simulink model "tyre"  (R2022b)
settings: Solver=ode4  StartTime=0.0  StopTime=simin.Time.data(end)  FixedStep=0.001  RelTol=1e-3
model workspace (MAT data in the model file):
  Fz_stat_FL = Simulink.Parameter
  Fz_stat_FL.Value = 3921.3656
  Fz_stat_FL.DataType = 'double'
  Fz_stat_FL.DocUnits = 'N'
  Fz_stat_FL.Complexity = 'real'
  Fz_stat_FL.Dimensions = [1 1]
  Fz_stat_FR = Simulink.Parameter
  Fz_stat_FR.Value = 3921.3656
  Fz_stat_FR.DataType = 'double'
  Fz_stat_FR.DocUnits = 'N'
  Fz_stat_FR.Complexity = 'real'
  Fz_stat_FR.Dimensions = [1 1]
  Fz_stat_RL = Simulink.Parameter
  Fz_stat_RL.Value = 3922.1269
  Fz_stat_RL.DataType = 'double'
  Fz_stat_RL.DocUnits = 'N'
  Fz_stat_RL.Complexity = 'real'
  Fz_stat_RL.Dimensions = [1 1]
  Fz_stat_RR = Simulink.Parameter
  Fz_stat_RR.Value = 3922.1267
  Fz_stat_RR.DataType = 'double'
  Fz_stat_RR.DocUnits = 'N'
  Fz_stat_RR.Complexity = 'real'
  Fz_stat_RR.Dimensions = [1 1]
  cog_height = Simulink.Parameter
  cog_height.Value = 0.604
  cog_height.DataType = 'double'
  cog_height.DocUnits = 'm'
  cog_height.Complexity = 'real'
  cog_height.Dimensions = [1 1]
  g = Simulink.Parameter
  g.Value = 9.806
  g.DataType = 'double'
  g.DocUnits = 'm/s^2'
  g.Complexity = 'real'
  g.Dimensions = [1 1]
  lF = Simulink.Parameter
  lF.Value = 1.466
  lF.DataType = 'double'
  lF.DocUnits = 'm'
  lF.Complexity = 'real'
  lF.Dimensions = [1 1]
  lR = Simulink.Parameter
  lR.Value = 1.509
  lR.DataType = 'double'
  lR.DocUnits = 'm'
  lR.Complexity = 'real'
  lR.Dimensions = [1 1]
  pitchAngle = Simulink.Parameter
  pitchAngle.Value = [0.00443372596055 0.00472012698538 0.00500652801021 0.00529292903504 0.00557933005986 0.00586573108469 0.00615213210952 0.00643853313435 0.00672493415917 0.007011335184 0.00729773620883 0.00758413723366 ... (200 elements, 1x200)]
  pitchAngle.DataType = 'double'
  pitchAngle.DocUnits = 'rad'
  pitchAngle.Complexity = 'real'
  pitchAngle.Dimensions = [1 200]
  pitchStiffness = Simulink.Parameter
  pitchStiffness.Value = [286621.759635 286644.842257 286407.773968 286374.136656 286600.567598 286901.705993 287109.32323 287190.659823 287245.018359 287344.728913 287488.533524 287631.863692 ... (200 elements, 1x200)]
  pitchStiffness.DataType = 'double'
  pitchStiffness.DocUnits = 'N*m*s/rad'
  pitchStiffness.Complexity = 'real'
  pitchStiffness.Dimensions = [1 200]
  pitch_inertia = Simulink.Parameter
  pitch_inertia.Value = 2180.5
  pitch_inertia.DataType = 'double'
  pitch_inertia.DocUnits = 'kg * m^2'
  pitch_inertia.Complexity = 'real'
  pitch_inertia.Dimensions = [1 1]
  pitching_coefficient = Simulink.Parameter
  pitching_coefficient.Value = -0.002
  pitching_coefficient.DataType = 'double'
  pitching_coefficient.DocUnits = '1'
  pitching_coefficient.Complexity = 'real'
  pitching_coefficient.Dimensions = [1 1]
  rdyn = Simulink.Parameter
  rdyn.Value = 0.309
  rdyn.DataType = 'double'
  rdyn.DocUnits = 'm'
  rdyn.Complexity = 'real'
  rdyn.Dimensions = [1 1]
  reference_area = Simulink.Parameter
  reference_area.Value = 2.4
  reference_area.DataType = 'double'
  reference_area.DocUnits = 'm^2'
  reference_area.Complexity = 'real'
  reference_area.Dimensions = [1 1]
  rho = Simulink.Parameter
  rho.Value = 1.2
  rho.DataType = 'double'
  rho.DocUnits = 'kg / m^3'
  rho.Complexity = 'real'
  rho.Dimensions = [1 1]
  rollStiffness_F = Simulink.Parameter
  rollStiffness_F.Value = -66168.4036
  rollStiffness_F.DataType = 'double'
  rollStiffness_F.DocUnits = 'N*m/rad'
  rollStiffness_F.Complexity = 'real'
  rollStiffness_F.Dimensions = [1 1]
  rollStiffness_R = Simulink.Parameter
  rollStiffness_R.Value = -79058.3706
  rollStiffness_R.DataType = 'double'
  rollStiffness_R.DocUnits = 'N*m/rad'
  rollStiffness_R.Complexity = 'real'
  rollStiffness_R.Dimensions = [1 1]
  sprung_mass = Simulink.Parameter
  sprung_mass.Value = 1373.3
  sprung_mass.DataType = 'double'
  sprung_mass.DocUnits = 'kg'
  sprung_mass.Complexity = 'real'
  sprung_mass.Dimensions = [1 1]
  tire = Simulink.Parameter
  tire.Value.MDI_Header.FILE_VERSION = 2
  tire.Value.Model.USE_MODE = 14
  tire.Value.Dim.UNLOADED_RADIUS = 0.3185
  tire.Value.Dim.WIDTH = 0.205
  tire.Value.Dim.RIM_RADIUS = 0.1905
  tire.Value.Dim.RIM_WIDTH = 0.1524
  tire.Value.Dim.ASPECT_RATIO = 0.6
  tire.Value.Vertical.VERTICAL_STIFFNESS = 236700
  tire.Value.Vertical.VERTICAL_DAMPING = 50
  tire.Value.Vertical.BREFF = 5
  tire.Value.Vertical.DREFF = 0.3
  tire.Value.Vertical.FREFF = 0.1
  tire.Value.Vertical.FNOMIN = 6500
  tire.Value.Range.KPUMIN = -0.3
  tire.Value.Range.KPUMAX = 0.3
  tire.Value.Range.ALPMIN = -0.1745
  tire.Value.Range.ALPMAX = 0.1745
  tire.Value.Range.CAMMIN = -0.1047
  tire.Value.Range.CAMMAX = 0.1047
  tire.Value.Range.FZMIN = 400
  tire.Value.Range.FZMAX = 8500
  tire.Value.Scale.LFZO = 1
  tire.Value.Scale.LCX = 1
  tire.Value.Scale.LMUX = 1
  tire.Value.Scale.LEX = 1
  tire.Value.Scale.LKX = 1
  tire.Value.Scale.LHX = 1
  tire.Value.Scale.LVX = 1
  tire.Value.Scale.LGAX = 1
  tire.Value.Scale.LCY = 1
  tire.Value.Scale.LMUY = 1
  tire.Value.Scale.LEY = 1
  tire.Value.Scale.LKY = 1
  tire.Value.Scale.LHY = 1
  tire.Value.Scale.LVY = 1
  tire.Value.Scale.LGAY = 1
  tire.Value.Scale.LTR = 1
  tire.Value.Scale.LRES = 1
  tire.Value.Scale.LGAZ = 1
  tire.Value.Scale.LXAL = 1
  tire.Value.Scale.LYKA = 1
  tire.Value.Scale.LVYKA = 1
  tire.Value.Scale.LS = 1
  tire.Value.Scale.LSGKP = 1
  tire.Value.Scale.LSGAL = 1
  tire.Value.Scale.LGYR = 1
  tire.Value.Scale.LMX = 1
  tire.Value.Scale.LVMX = 1
  tire.Value.Scale.LMY = 1
  tire.Value.Long.PCX1 = 1.6055
  tire.Value.Long.PDX1 = 1.1703
  tire.Value.Long.PDX2 = -0.081328
  tire.Value.Long.PDX3 = 0
  tire.Value.Long.PEX1 = 0.53409
  tire.Value.Long.PEX2 = -0.019956
  tire.Value.Long.PEX3 = 0.18089
  tire.Value.Long.PEX4 = 2.9951e-07
  tire.Value.Long.PKX1 = 36.411
  tire.Value.Long.PKX2 = 0.12615
  tire.Value.Long.PKX3 = 0.51289
  tire.Value.Long.PHX1 = 0
  tire.Value.Long.PHX2 = 0
  tire.Value.Long.PVX1 = 0
  tire.Value.Long.PVX2 = 0
  tire.Value.Long.RBX1 = 18.456
  tire.Value.Long.RBX2 = 16.314
  tire.Value.Long.RCX1 = 1.091
  tire.Value.Long.REX1 = 0
  tire.Value.Long.REX2 = 0
  tire.Value.Long.RHX1 = 0.0058715
  tire.Value.Long.PTX1 = 1.5
  tire.Value.Long.PTX2 = 0.180096
  tire.Value.Long.PTX3 = -0.15
  tire.Value.OverTurn.QSX1 = 0.00023155
  tire.Value.OverTurn.QSX2 = 0.51574
  tire.Value.OverTurn.QSX3 = 0.046399
  tire.Value.Lat.PCY1 = 2.1322
  tire.Value.Lat.PDY1 = 1.0283
  tire.Value.Lat.PDY2 = -0.16758
  tire.Value.Lat.PDY3 = -1.5821
  tire.Value.Lat.PEY1 = 0.33443
  tire.Value.Lat.PEY2 = -1.8733
  tire.Value.Lat.PEY3 = -0.13136
  tire.Value.Lat.PEY4 = -11.677
  tire.Value.Lat.PKY1 = -20.505
  tire.Value.Lat.PKY2 = 2.0284
  tire.Value.Lat.PKY3 = 0.89994
  tire.Value.Lat.PHY1 = 0.0031377
  tire.Value.Lat.PHY2 = 0.00051596
  tire.Value.Lat.PHY3 = 0.039251
  tire.Value.Lat.PVY1 = 0.026365
  tire.Value.Lat.PVY2 = -0.0062119
  tire.Value.Lat.PVY3 = -0.41389
  tire.Value.Lat.PVY4 = -0.048038
  tire.Value.Lat.RBY1 = 22.003
  tire.Value.Lat.RBY2 = -13.623
  tire.Value.Lat.RBY3 = -0.0093616
  tire.Value.Lat.RCY1 = 0.98294
  tire.Value.Lat.REY1 = 0
  tire.Value.Lat.REY2 = 0
  tire.Value.Lat.RHY1 = -9.1492e-11
  tire.Value.Lat.RHY2 = 0
  tire.Value.Lat.RVY1 = 22.965
  tire.Value.Lat.RVY2 = 0.37981
  tire.Value.Lat.RVY3 = 1.8552
  tire.Value.Lat.RVY4 = 0.08767
  tire.Value.Lat.RVY5 = -8.8234e-11
  tire.Value.Lat.RVY6 = 0.90374
  tire.Value.Lat.PTY1 = 1.75
  tire.Value.Lat.PTY2 = 1.35
  tire.Value.Roll.QSY1 = 0.01
  tire.Value.Roll.QSY2 = 0
  tire.Value.Roll.QSY3 = 0
  tire.Value.Roll.QSY4 = 0
  tire.Value.Align.QBZ1 = 19.588
  tire.Value.Align.QBZ2 = -4.1671
  tire.Value.Align.QBZ3 = -0.34132
  tire.Value.Align.QBZ4 = -0.023607
  tire.Value.Align.QBZ5 = -0.0793
  tire.Value.Align.QBZ9 = -50
  tire.Value.Align.QBZ10 = 0
  tire.Value.Align.QCZ1 = 1.2012
  tire.Value.Align.QDZ1 = 0.12819
  tire.Value.Align.QDZ2 = -0.0052433
  tire.Value.Align.QDZ3 = -0.099544
  tire.Value.Align.QDZ4 = -15
  tire.Value.Align.QDZ6 = 6.2499e-05
  tire.Value.Align.QDZ7 = 0.00050135
  tire.Value.Align.QDZ8 = -0.28564
  tire.Value.Align.QDZ9 = -0.025056
  tire.Value.Align.QEZ1 = -0.0044308
  tire.Value.Align.QEZ2 = 0.022579
  tire.Value.Align.QEZ3 = -0.16199
  tire.Value.Align.QEZ4 = -0.5576
  tire.Value.Align.QEZ5 = -87.296
  tire.Value.Align.QHZ1 = 0.00082436
  tire.Value.Align.QHZ2 = 0.002733
  tire.Value.Align.QHZ3 = 0.15
  tire.Value.Align.QHZ4 = 0.11608
  tire.Value.Align.SSZ1 = -5.3899e-10
  tire.Value.Align.SSZ2 = -2.2371e-09
  tire.Value.Align.SSZ3 = 3.6029e-08
  tire.Value.Align.SSZ4 = 3.9826e-08
  tire.Value.Align.QTZ1 = 0.3
  tire.Value.Align.MBELT = 7.5
  tire.Value.FLoadMax = 10000
  tire.DataType = 'struct'
  tire.Complexity = 'real'
  tire.Dimensions = [1 1]
  total_pitchDamping = Simulink.Parameter
  total_pitchDamping.Value = 22000
  total_pitchDamping.DataType = 'double'
  total_pitchDamping.DocUnits = 'N*m/rad'
  total_pitchDamping.Complexity = 'real'
  total_pitchDamping.Dimensions = [1 1]
  total_pitchStiffness = Simulink.Parameter
  total_pitchStiffness.Value = 291158.1055
  total_pitchStiffness.DataType = 'double'
  total_pitchStiffness.DocUnits = 'N*m/rad'
  total_pitchStiffness.Complexity = 'real'
  total_pitchStiffness.Dimensions = [1 1]
  total_rollStiffness = Simulink.Parameter
  total_rollStiffness.Value = 138201.9734
  total_rollStiffness.DataType = 'double'
  total_rollStiffness.DocUnits = 'N*m/rad'
  total_rollStiffness.Complexity = 'real'
  total_rollStiffness.Dimensions = [1 1]
  trackwidth_F = Simulink.Parameter
  trackwidth_F.Value = 1.6
  trackwidth_F.DataType = 'double'
  trackwidth_F.DocUnits = 'm'
  trackwidth_F.Complexity = 'real'
  trackwidth_F.Dimensions = [1 1]
  trackwidth_R = Simulink.Parameter
  trackwidth_R.Value = 1.614
  trackwidth_R.DataType = 'double'
  trackwidth_R.DocUnits = 'm'
  trackwidth_R.Complexity = 'real'
  trackwidth_R.Dimensions = [1 1]
  unsprung_mass = Simulink.Parameter
  unsprung_mass.Value = 226.704
  unsprung_mass.DataType = 'double'
  unsprung_mass.DocUnits = 'kg'
  unsprung_mass.Complexity = 'real'
  unsprung_mass.Dimensions = [1 1]
  wheelbase = Simulink.Parameter
  wheelbase.Value = 2.975
  wheelbase.DataType = 'double'
  wheelbase.DocUnits = 'm'
  wheelbase.Complexity = 'real'
  wheelbase.Dimensions = [1 1]
values from neighbouring files (symbols this model uses):
  lF = Simulink.Parameter    [controller_2022b_saveas.m]
  lR = Simulink.Parameter    [controller_2022b_saveas.m]
  tire = Simulink.Parameter    [controller_2022b_saveas.m]
  trackwidth_F = Simulink.Parameter    [controller_2022b_saveas.m]
  trackwidth_R = Simulink.Parameter    [controller_2022b_saveas.m]
undefined symbols (not defined in the file or in its folder): DiscIntNeverNeededParam
settings Model: Creator=marcel  LastModifiedBy=marce

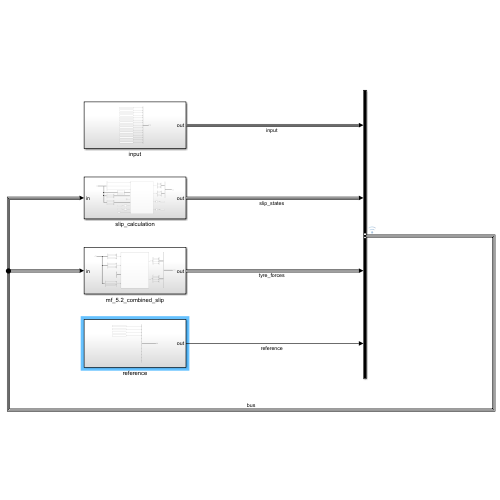
[thumbnail: Simulink's stored preview of the top-level diagram]
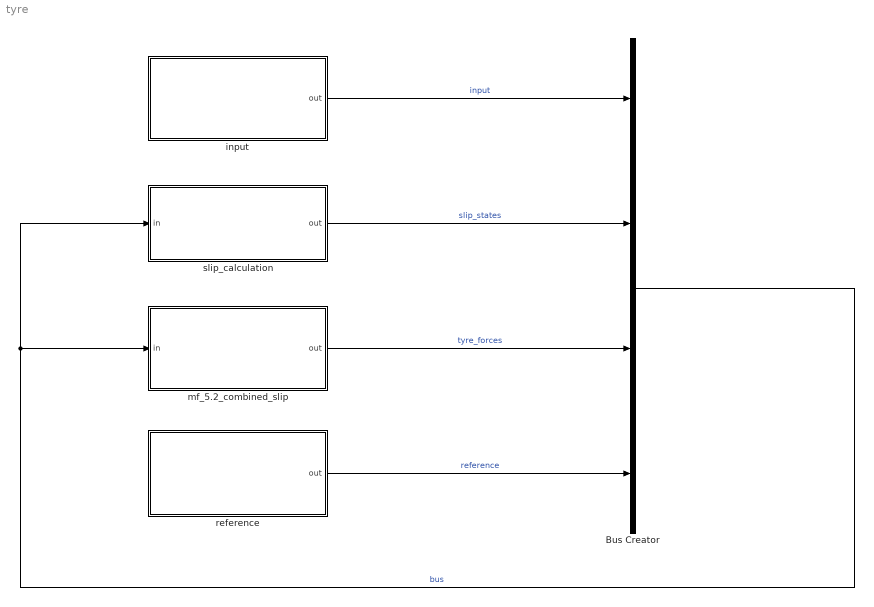
== system tyre ==
  Bus Creator : BusCreator  Inputs=4
  input : Subsystem
  mf_5.2_combined_slip : Subsystem
  reference : Subsystem
  slip_calculation : Subsystem
  wires:
  input/1(out) -> Bus Creator/1  "input"
  slip_calculation/1(out) -> Bus Creator/2  "slip_states"
  mf_5.2_combined_slip/1(out) -> Bus Creator/3  "tyre_forces"
  Bus Creator/1 -> mf_5.2_combined_slip/1(in), slip_calculation/1(in)  "bus"
  reference/1(out) -> Bus Creator/4  "reference"

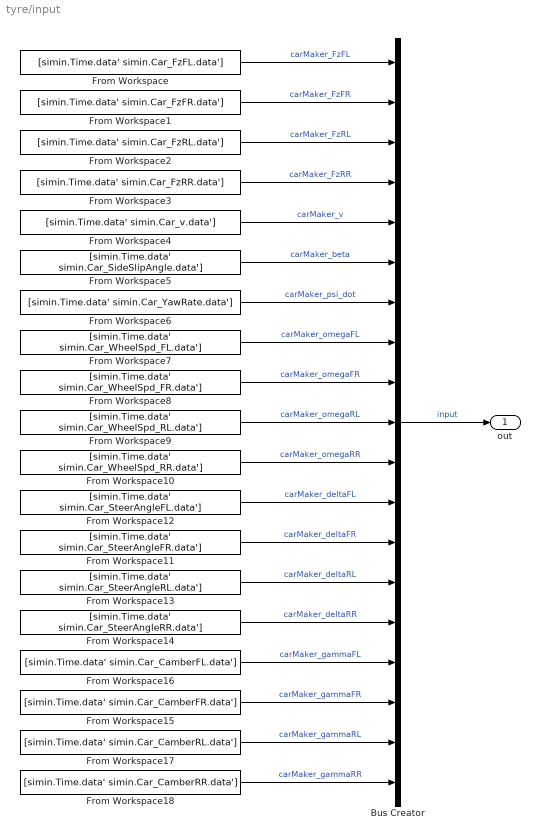
== system tyre/input ==
  Bus Creator : BusCreator  Inputs=19
  From Workspace : FromWorkspace  VariableName=[simin.Time.data' simin.Car_FzFL.data']
  From Workspace1 : FromWorkspace  VariableName=[simin.Time.data' simin.Car_FzFR.data']
  From Workspace10 : FromWorkspace  VariableName=[simin.Time.data' simin.Car_WheelSpd_RR.data']
  From Workspace11 : FromWorkspace  VariableName=[simin.Time.data' simin.Car_SteerAngleFR.data']
  From Workspace12 : FromWorkspace  VariableName=[simin.Time.data' simin.Car_SteerAngleFL.data']
  From Workspace13 : FromWorkspace  VariableName=[simin.Time.data' simin.Car_SteerAngleRL.data']
  From Workspace14 : FromWorkspace  VariableName=[simin.Time.data' simin.Car_SteerAngleRR.data']
  From Workspace15 : FromWorkspace  VariableName=[simin.Time.data' simin.Car_CamberFR.data']
  From Workspace16 : FromWorkspace  VariableName=[simin.Time.data' simin.Car_CamberFL.data']
  From Workspace17 : FromWorkspace  VariableName=[simin.Time.data' simin.Car_CamberRL.data']
  From Workspace18 : FromWorkspace  VariableName=[simin.Time.data' simin.Car_CamberRR.data']
  From Workspace2 : FromWorkspace  VariableName=[simin.Time.data' simin.Car_FzRL.data']
  From Workspace3 : FromWorkspace  VariableName=[simin.Time.data' simin.Car_FzRR.data']
  From Workspace4 : FromWorkspace  VariableName=[simin.Time.data' simin.Car_v.data']
  From Workspace5 : FromWorkspace  VariableName=[simin.Time.data' simin.Car_SideSlipAngle.data']
  From Workspace6 : FromWorkspace  VariableName=[simin.Time.data' simin.Car_YawRate.data']
  From Workspace7 : FromWorkspace  VariableName=[simin.Time.data' simin.Car_WheelSpd_FL.data']
  From Workspace8 : FromWorkspace  VariableName=[simin.Time.data' simin.Car_WheelSpd_FR.data']
  From Workspace9 : FromWorkspace  VariableName=[simin.Time.data' simin.Car_WheelSpd_RL.data']
  out : Outport
  wires:
  Bus Creator/1 -> out/1  "input"
  From Workspace/1 -> Bus Creator/1  "carMaker_FzFL"
  From Workspace1/1 -> Bus Creator/2  "carMaker_FzFR"
  From Workspace2/1 -> Bus Creator/3  "carMaker_FzRL"
  From Workspace3/1 -> Bus Creator/4  "carMaker_FzRR"
  From Workspace4/1 -> Bus Creator/5  "carMaker_v"
  From Workspace5/1 -> Bus Creator/6  "carMaker_beta"
  From Workspace6/1 -> Bus Creator/7  "carMaker_psi_dot"
  From Workspace7/1 -> Bus Creator/8  "carMaker_omegaFL"
  From Workspace8/1 -> Bus Creator/9  "carMaker_omegaFR"
  From Workspace9/1 -> Bus Creator/10  "carMaker_omegaRL"
  From Workspace10/1 -> Bus Creator/11  "carMaker_omegaRR"
  From Workspace12/1 -> Bus Creator/12  "carMaker_deltaFL"
  From Workspace11/1 -> Bus Creator/13  "carMaker_deltaFR"
  From Workspace13/1 -> Bus Creator/14  "carMaker_deltaRL"
  From Workspace14/1 -> Bus Creator/15  "carMaker_deltaRR"
  From Workspace16/1 -> Bus Creator/16  "carMaker_gammaFL"
  From Workspace15/1 -> Bus Creator/17  "carMaker_gammaFR"
  From Workspace17/1 -> Bus Creator/18  "carMaker_gammaRL"
  From Workspace18/1 -> Bus Creator/19  "carMaker_gammaRR"

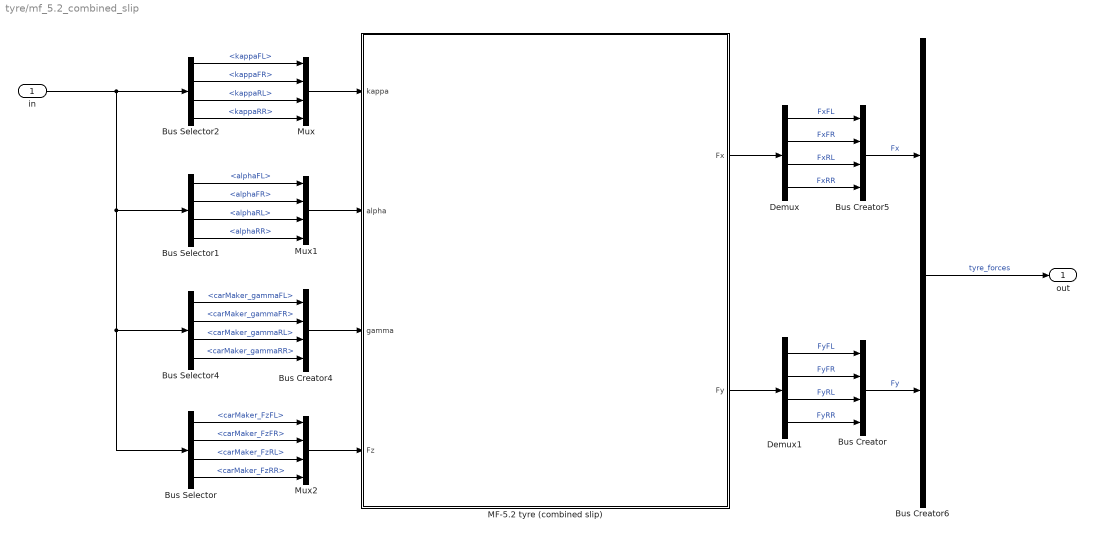
== system tyre/mf_5.2_combined_slip ==
  in : Inport
  Bus Creator : BusCreator  Inputs=4
  Bus Creator4 : BusCreator  Inputs=4
  Bus Creator5 : BusCreator  Inputs=4
  Bus Creator6 : BusCreator  Inputs=2
  Bus Selector : BusSelector  OutputSignals=input.carMaker_FzFL,input.carMaker_FzFR,input.carMaker_FzRL,input.carMaker_FzRR
  Bus Selector1 : BusSelector  OutputSignals=slip_states.alpha.alphaFL,slip_states.alpha.alphaFR,slip_states.alpha.alphaRL,slip_states.alpha.alphaRR
  Bus Selector2 : BusSelector  OutputSignals=slip_states.kappa.kappaFL,slip_states.kappa.kappaFR,slip_states.kappa.kappaRL,slip_states.kappa.kappaRR
  Bus Selector4 : BusSelector  OutputSignals=input.carMaker_gammaFL,input.carMaker_gammaFR,input.carMaker_gammaRL,input.carMaker_gammaRR
  Demux : Demux
  Demux1 : Demux
  MF-5.2 tyre (combined slip) : MATLAB Function  TreatAsAtomicUnit=on
  Mux : Mux
  Mux1 : Mux
  Mux2 : Mux
  out : Outport
  wires:
  MF-5.2 tyre (combined slip)/1(Fx) -> Demux/1
  Bus Creator4/1 -> MF-5.2 tyre (combined slip)/3(gamma)
  Bus Selector/4 -> Mux2/4  "<carMaker_FzRR>"
  Bus Selector/3 -> Mux2/3  "<carMaker_FzRL>"
  Mux2/1 -> MF-5.2 tyre (combined slip)/4(Fz)
  Bus Selector/1 -> Mux2/1  "<carMaker_FzFL>"
  Bus Selector/2 -> Mux2/2  "<carMaker_FzFR>"
  Bus Selector1/1 -> Mux1/1  "<alphaFL>"
  Bus Selector1/2 -> Mux1/2  "<alphaFR>"
  Bus Selector1/3 -> Mux1/3  "<alphaRL>"
  Bus Selector1/4 -> Mux1/4  "<alphaRR>"
  Mux1/1 -> MF-5.2 tyre (combined slip)/2(alpha)
  Mux/1 -> MF-5.2 tyre (combined slip)/1(kappa)
  Bus Selector2/1 -> Mux/1  "<kappaFL>"
  Bus Selector2/2 -> Mux/2  "<kappaFR>"
  Bus Selector2/3 -> Mux/3  "<kappaRL>"
  Bus Selector2/4 -> Mux/4  "<kappaRR>"
  MF-5.2 tyre (combined slip)/2(Fy) -> Demux1/1
  Demux1/1 -> Bus Creator/1  "FyFL"
  Demux1/2 -> Bus Creator/2  "FyFR"
  Demux1/3 -> Bus Creator/3  "FyRL"
  Demux1/4 -> Bus Creator/4  "FyRR"
  Demux/1 -> Bus Creator5/1  "FxFL"
  Demux/2 -> Bus Creator5/2  "FxFR"
  Demux/3 -> Bus Creator5/3  "FxRL"
  Demux/4 -> Bus Creator5/4  "FxRR"
  Bus Creator/1 -> Bus Creator6/2  "Fy"
  Bus Creator5/1 -> Bus Creator6/1  "Fx"
  Bus Creator6/1 -> out/1  "tyre_forces"
  Bus Selector4/1 -> Bus Creator4/1  "<carMaker_gammaFL>"
  in/1 -> Bus Selector1/1, Bus Selector4/1, Bus Selector/1, Bus Selector2/1
  Bus Selector4/2 -> Bus Creator4/2  "<carMaker_gammaFR>"
  Bus Selector4/3 -> Bus Creator4/3  "<carMaker_gammaRL>"
  Bus Selector4/4 -> Bus Creator4/4  "<carMaker_gammaRR>"

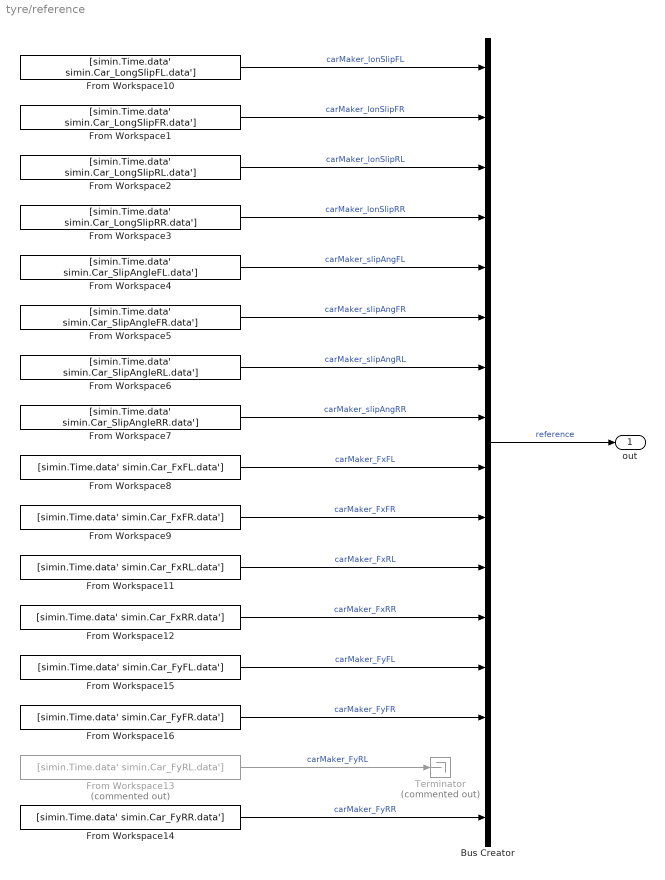
== system tyre/reference ==
  Bus Creator : BusCreator  Inputs=16
  From Workspace1 : FromWorkspace  VariableName=[simin.Time.data' simin.Car_LongSlipFR.data']
  From Workspace10 : FromWorkspace  VariableName=[simin.Time.data' simin.Car_LongSlipFL.data']
  From Workspace11 : FromWorkspace  VariableName=[simin.Time.data' simin.Car_FxRL.data']
  From Workspace12 : FromWorkspace  VariableName=[simin.Time.data' simin.Car_FxRR.data']
  From Workspace13 : FromWorkspace  Commented=on  VariableName=[simin.Time.data' simin.Car_FyRL.data']
  From Workspace14 : FromWorkspace  VariableName=[simin.Time.data' simin.Car_FyRR.data']
  From Workspace15 : FromWorkspace  VariableName=[simin.Time.data' simin.Car_FyFL.data']
  From Workspace16 : FromWorkspace  VariableName=[simin.Time.data' simin.Car_FyFR.data']
  From Workspace2 : FromWorkspace  VariableName=[simin.Time.data' simin.Car_LongSlipRL.data']
  From Workspace3 : FromWorkspace  VariableName=[simin.Time.data' simin.Car_LongSlipRR.data']
  From Workspace4 : FromWorkspace  VariableName=[simin.Time.data' simin.Car_SlipAngleFL.data']
  From Workspace5 : FromWorkspace  VariableName=[simin.Time.data' simin.Car_SlipAngleFR.data']
  From Workspace6 : FromWorkspace  VariableName=[simin.Time.data' simin.Car_SlipAngleRL.data']
  From Workspace7 : FromWorkspace  VariableName=[simin.Time.data' simin.Car_SlipAngleRR.data']
  From Workspace8 : FromWorkspace  VariableName=[simin.Time.data' simin.Car_FxFL.data']
  From Workspace9 : FromWorkspace  VariableName=[simin.Time.data' simin.Car_FxFR.data']
  Terminator : Terminator  Commented=on
  out : Outport
  wires:
  Bus Creator/1 -> out/1  "reference"
  From Workspace10/1 -> Bus Creator/1  "carMaker_lonSlipFL"
  From Workspace1/1 -> Bus Creator/2  "carMaker_lonSlipFR"
  From Workspace2/1 -> Bus Creator/3  "carMaker_lonSlipRL"
  From Workspace3/1 -> Bus Creator/4  "carMaker_lonSlipRR"
  From Workspace4/1 -> Bus Creator/5  "carMaker_slipAngFL"
  From Workspace5/1 -> Bus Creator/6  "carMaker_slipAngFR"
  From Workspace6/1 -> Bus Creator/7  "carMaker_slipAngRL"
  From Workspace7/1 -> Bus Creator/8  "carMaker_slipAngRR"
  From Workspace12/1 -> Bus Creator/12  "carMaker_FxRR"
  From Workspace11/1 -> Bus Creator/11  "carMaker_FxRL"
  From Workspace9/1 -> Bus Creator/10  "carMaker_FxFR"
  From Workspace8/1 -> Bus Creator/9  "carMaker_FxFL"
  From Workspace15/1 -> Bus Creator/13  "carMaker_FyFL"
  From Workspace16/1 -> Bus Creator/14  "carMaker_FyFR"
  From Workspace13/1 -> Terminator/1  "carMaker_FyRL"
  From Workspace14/1 -> Bus Creator/16  "carMaker_FyRR"

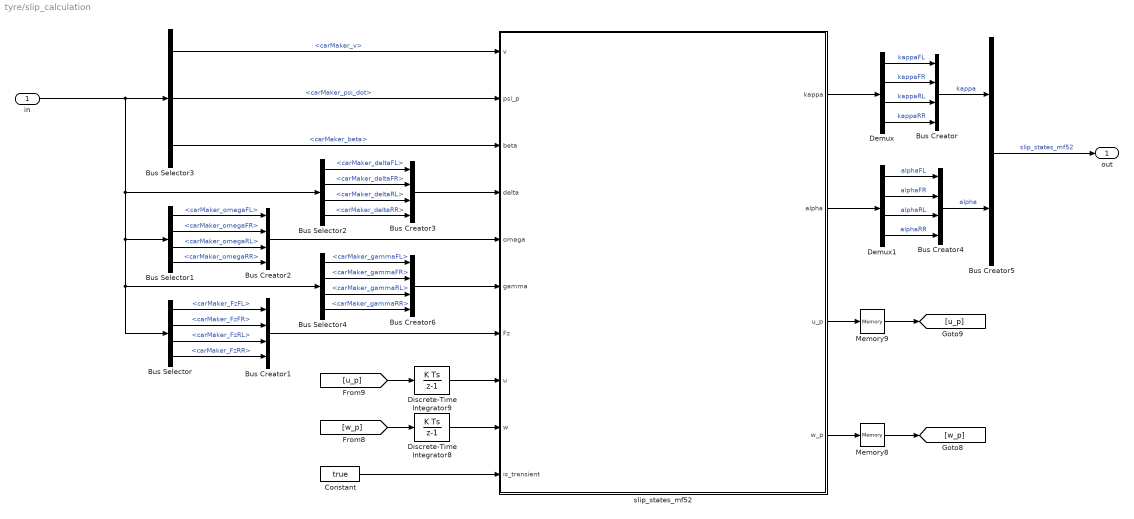
== system tyre/slip_calculation ==
  in : Inport
  Bus Creator{,1..4,6} (6 alike) : BusCreator  Inputs=4
  Bus Creator5 : BusCreator  Inputs=2
  Bus Selector : BusSelector  OutputSignals=input.carMaker_FzFL,input.carMaker_FzFR,input.carMaker_FzRL,input.carMaker_FzRR
  Bus Selector1 : BusSelector  OutputSignals=input.carMaker_omegaFL,input.carMaker_omegaFR,input.carMaker_omegaRL,input.carMaker_omegaRR
  Bus Selector2 : BusSelector  OutputSignals=input.carMaker_deltaFL,input.carMaker_deltaFR,input.carMaker_deltaRL,input.carMaker_deltaRR
  Bus Selector3 : BusSelector  OutputSignals=input.carMaker_v,input.carMaker_psi_dot,input.carMaker_beta
  Bus Selector4 : BusSelector  OutputSignals=input.carMaker_gammaFL,input.carMaker_gammaFR,input.carMaker_gammaRL,input.carMaker_gammaRR
  Constant : Constant  Value=true  OutDataTypeStr=boolean
  Demux : Demux
  Demux1 : Demux
  Discrete-Time Integrator8 : DiscreteIntegrator  SampleTime=-1  UpperSaturationLimit=0.1  LowerSaturationLimit=-0.1  ICPrevOutput=DiscIntNeverNeededParam  ICPrevScaledInput=DiscIntNeverNeededParam
  Discrete-Time Integrator9 : DiscreteIntegrator  SampleTime=-1  UpperSaturationLimit=0.01  LowerSaturationLimit=-0.01  ICPrevOutput=DiscIntNeverNeededParam  ICPrevScaledInput=DiscIntNeverNeededParam
  Memory8 : Memory
  Memory9 : Memory
  slip_states_mf52 : MATLAB Function  TreatAsAtomicUnit=on
  out : Outport
  wires:
  in/1 -> Bus Selector2/1, Bus Selector1/1, Bus Selector4/1, Bus Selector/1, Bus Selector3/1
  Discrete-Time Integrator8/1 -> slip_states_mf52/9(w)
  [w_p] -> Discrete-Time Integrator8/1
  Bus Creator6/1 -> slip_states_mf52/6(gamma)
  Discrete-Time Integrator9/1 -> slip_states_mf52/8(u)
  slip_states_mf52/3(u_p) -> Memory9/1
  Memory8/1 -> [w_p]
  Constant/1 -> slip_states_mf52/10(is_transient)
  slip_states_mf52/4(w_p) -> Memory8/1
  Bus Creator2/1 -> slip_states_mf52/5(omega)
  Memory9/1 -> [u_p]
  [u_p] -> Discrete-Time Integrator9/1
  Bus Creator1/1 -> slip_states_mf52/7(Fz)
  Bus Selector/1 -> Bus Creator1/1  "<carMaker_FzFL>"
  Bus Selector/2 -> Bus Creator1/2  "<carMaker_FzFR>"
  Bus Selector/3 -> Bus Creator1/3  "<carMaker_FzRL>"
  Bus Selector/4 -> Bus Creator1/4  "<carMaker_FzRR>"
  Bus Selector1/1 -> Bus Creator2/1  "<carMaker_omegaFL>"
  Bus Selector1/2 -> Bus Creator2/2  "<carMaker_omegaFR>"
  Bus Selector1/3 -> Bus Creator2/3  "<carMaker_omegaRL>"
  Bus Selector1/4 -> Bus Creator2/4  "<carMaker_omegaRR>"
  Bus Creator3/1 -> slip_states_mf52/4(delta)
  Bus Selector2/4 -> Bus Creator3/4  "<carMaker_deltaRR>"
  Bus Selector2/3 -> Bus Creator3/3  "<carMaker_deltaRL>"
  Bus Selector2/2 -> Bus Creator3/2  "<carMaker_deltaFR>"
  Bus Selector2/1 -> Bus Creator3/1  "<carMaker_deltaFL>"
  Bus Selector3/1 -> slip_states_mf52/1(v)  "<carMaker_v>"
  Bus Selector3/3 -> slip_states_mf52/3(beta)  "<carMaker_beta>"
  Bus Selector3/2 -> slip_states_mf52/2(psi_p)  "<carMaker_psi_dot>"
  slip_states_mf52/1(kappa) -> Demux/1
  slip_states_mf52/2(alpha) -> Demux1/1
  Demux/1 -> Bus Creator/1  "kappaFL"
  Demux/2 -> Bus Creator/2  "kappaFR"
  Demux/3 -> Bus Creator/3  "kappaRL"
  Demux/4 -> Bus Creator/4  "kappaRR"
  Demux1/4 -> Bus Creator4/4  "alphaRR"
  Demux1/2 -> Bus Creator4/2  "alphaFR"
  Demux1/3 -> Bus Creator4/3  "alphaRL"
  Demux1/1 -> Bus Creator4/1  "alphaFL"
  Bus Creator4/1 -> Bus Creator5/2  "alpha"
  Bus Creator/1 -> Bus Creator5/1  "kappa"
  Bus Creator5/1 -> out/1  "slip_states_mf52"
  Bus Selector4/1 -> Bus Creator6/1  "<carMaker_gammaFL>"
  Bus Selector4/2 -> Bus Creator6/2  "<carMaker_gammaFR>"
  Bus Selector4/3 -> Bus Creator6/3  "<carMaker_gammaRL>"
  Bus Selector4/4 -> Bus Creator6/4  "<carMaker_gammaRR>"

== matlab function tyre/mf_5.2_combined_slip/MF-5.2 tyre (combined slip) ==
  data: kappa input size=[4]; alpha input size=[4]; gamma input size=[4]; Fz input size=[4]; Fx output size=[1 4]; tire parameter; Fy output size=[1 4]
function [Fx, Fy] = fcn(kappa, alpha, gamma, Fz, tire)
    %% determine output sizes
    % step is needed so simulink now the sizes when compiling
    % Fx = zeros(1,4);
    % Fy = zeros(1,4);

    %% parameter mapping

    % vertical
    F_z0 = tire.Vertical.FNOMIN;

    % longitudinal (pure slip)
    p_Cx1 = tire.Long.PCX1;
    
    p_Dx1 = tire.Long.PDX1; 
    p_Dx2 = tire.Long.PDX2;
    p_Dx3 = tire.Long.PDX3;
    
    p_Ex1 = tire.Long.PEX1;
    p_Ex2 = tire.Long.PEX2;
    p_Ex3 = tire.Long.PEX3;
    p_Ex4 = tire.Long.PEX4;
    
    p_Kx1 = tire.Long.PKX1;
    p_Kx2 = tire.Long.PKX2;
    p_Kx3 = tire.Long.PKX3;
    
    p_Hx1 = tire.Long.PHX1;
    p_Hx2 = tire.Long.PHX2;
    
    p_Vx1 = tire.Long.PVX1;
    p_Vx2 = tire.Long.PVX2;
    
    % lateral (pure slip)
    p_Cy1 = tire.Lat.PCY1;
    
    p_Dy1 = tire.Lat.PDY1;
    p_Dy2 = tire.Lat.PDY2;
    p_Dy3 = tire.Lat.PDY3;
    
    p_Ey1 = tire.Lat.PEY1;
    p_Ey2 = tire.Lat.PEY2;
    p_Ey3 = tire.Lat.PEY3;
    p_Ey4 = tire.Lat.PEY4;
    
    p_Ky1 = tire.Lat.PKY1;
    p_Ky2 = tire.Lat.PKY2;
    p_Ky3 = tire.Lat.PKY3;
    
    p_Hy1 = tire.Lat.PHY1;
    p_Hy2 = tire.Lat.PHY2;
    p_Hy3 = tire.Lat.PHY3;
    
    p_Vy1 = tire.Lat.PVY1;
    p_Vy2 = tire.Lat.PVY2;
    p_Vy3 = tire.Lat.PVY3;
    p_Vy4 = tire.Lat.PVY4;
    
    % longitudinal (combined slip)
    r_Bx1 = tire.Long.RBX1;
    r_Bx2 = tire.Long.RBX2;
    
    r_Cx1 = tire.Long.RCX1;
    
    r_Ex1 = tire.Long.REX1;
    r_Ex2 = tire.Long.REX2;
    
    r_Hx1 = tire.Long.RHX1;
    
    % lateral (combined slip)
    r_By1 = tire.Lat.RBY1;
    r_By2 = tire.Lat.RBY2;
    r_By3 = tire.Lat.RBY3;
    
    r_Cy1 = tire.Lat.RCY1;
    
    r_Ey1 = tire.Lat.REY1;
    r_Ey2 = tire.Lat.REY2;
    
    r_Hy1 = tire.Lat.RHY1;
    r_Hy2 = tire.Lat.RHY2;
    
    r_Vy1 = tire.Lat.RVY1;
    r_Vy2 = tire.Lat.RVY2;
    r_Vy3 = tire.Lat.RVY3;
    r_Vy4 = tire.Lat.RVY4;
    r_Vy5 = tire.Lat.RVY5;
    r_Vy6 = tire.Lat.RVY6;

    %% vertical load mapping
    Fz_FL = Fz(1);
    Fz_FR = Fz(2);
    Fz_RL = Fz(3);
    Fz_RR = Fz(4);

    %% longitudinal slip mapping
    long_slip_FL = kappa(1);
    long_slip_FR = kappa(2);
    long_slip_RL = kappa(3);
    long_slip_RR = kappa(4);

    %% side slip angle mapping
    slip_ang_FL = alpha(1);
    slip_ang_FR = alpha(2);
    slip_ang_RL = alpha(3);
    slip_ang_RR = alpha(4);

    %% camber vector
    gamma_FL = gamma(1);
    gamma_FR = gamma(2);
    gamma_RL = gamma(3);
    gamma_RR = gamma(4);

    %% normalized vertical load
    % equations from Delft MF-Tyre User Manual Version 5.2
    % page 17
    dfz_FL = (Fz_FL - F_z0) / F_z0;
    dfz_FR = (Fz_FR - F_z0) / F_z0; 
    dfz_RL = (Fz_RL - F_z0) / F_z0; 
    dfz_RR = (Fz_RR - F_z0) / F_z0;

    %% longitudinal (pure slip)
    % equations from Delft MF-Tyre User Manual Version 5.2
    % page 22 - 24
    Cx = p_Cx1; % - each wheel is equipped with the same tyre
    
    mu_x_FL = (p_Dx1 + p_Dx2 .* dfz_FL) .* (1 - p_Dx3 .* gamma_FL.^2);
    mu_x_FR = (p_Dx1 + p_Dx2 .* dfz_FR) .* (1 - p_Dx3 .* gamma_FR.^2);
    mu_x_RL = (p_Dx1 + p_Dx2 .* dfz_RL) .* (1 - p_Dx3 .* gamma_RL.^2);
    mu_x_RR = (p_Dx1 + p_Dx2 .* dfz_RR) .* (1 - p_Dx3 .* gamma_RR.^2);

    Dx_FL = mu_x_FL .* Fz_FL;
    Dx_FR = mu_x_FR .* Fz_FR;
    Dx_RL = mu_x_RL .* Fz_RL;
    Dx_RR = mu_x_RR .* Fz_RR;
    
    S_Hx_FL = (p_Hx1 + p_Hx2 .* dfz_FL);
    S_Hx_FR = (p_Hx1 + p_Hx2 .* dfz_FR);
    S_Hx_RL = (p_Hx1 + p_Hx2 .* dfz_RL);
    S_Hx_RR = (p_Hx1 + p_Hx2 .* dfz_RR);

    S_Vx_FL = Fz_FL .* (p_Vx1 + p_Vx2 .* dfz_FL);
    S_Vx_FR = Fz_FR .* (p_Vx1 + p_Vx2 .* dfz_FR);
    S_Vx_RL = Fz_RL .* (p_Vx1 + p_Vx2 .* dfz_RL);
    S_Vx_RR = Fz_RR .* (p_Vx1 + p_Vx2 .* dfz_RR);
    
    kappa_x_FL = long_slip_FL + S_Hx_FL;
    kappa_x_FR = long_slip_FR + S_Hx_FR;
    kappa_x_RL = long_slip_RL + S_Hx_RL;
    kappa_x_RR = long_slip_RR + S_Hx_RR;
    
    Ex_FL = (p_Ex1 + p_Ex2 .* dfz_FL + p_Ex3 .* dfz_FL.^2) .* (1 - p_Ex4 .* sign(kappa_x_FL));
    Ex_FR = (p_Ex1 + p_Ex2 .* dfz_FR + p_Ex3 .* dfz_FR.^2) .* (1 - p_Ex4 .* sign(kappa_x_FR));
    Ex_RL = (p_Ex1 + p_Ex2 .* dfz_RL + p_Ex3 .* dfz_RL.^2) .* (1 - p_Ex4 .* sign(kappa_x_RL));
    Ex_RR = (p_Ex1 + p_Ex2 .* dfz_RR + p_Ex3 .* dfz_RR.^2) .* (1 - p_Ex4 .* sign(kappa_x_RR));

    Kx_FL = Fz_FL .* (p_Kx1 + p_Kx2 .* dfz_FL) .* exp(p_Kx3 .* dfz_FL);
    Kx_FR = Fz_FR .* (p_Kx1 + p_Kx2 .* dfz_FR) .* exp(p_Kx3 .* dfz_FR);
    Kx_RL = Fz_RL .* (p_Kx1 + p_Kx2 .* dfz_RL) .* exp(p_Kx3 .* dfz_RL);
    Kx_RR = Fz_RR .* (p_Kx1 + p_Kx2 .* dfz_RR) .* exp(p_Kx3 .* dfz_RR);

    Bx_FL = Kx_FL ./ (Cx .* Dx_FL);
    Bx_FR = Kx_FR ./ (Cx .* Dx_FR);
    Bx_RL = Kx_RL ./ (Cx .* Dx_RL);
    Bx_RR = Kx_RR ./ (Cx .* Dx_RR);
    
    Fx0_FL = Dx_FL .* sin(Cx .* atan(Bx_FL .* kappa_x_FL - Ex_FL .* (Bx_FL .* kappa_x_FL - atan(Bx_FL .* kappa_x_FL)))) + S_Vx_FL; % will later be used in combined slip equations
    Fx0_FR = Dx_FR .* sin(Cx .* atan(Bx_FR .* kappa_x_FR - Ex_FR .* (Bx_FR .* kappa_x_FR - atan(Bx_FR .* kappa_x_FR)))) + S_Vx_FR; % will later be used in combined slip equations
    Fx0_RL = Dx_RL .* sin(Cx .* atan(Bx_RL .* kappa_x_RL - Ex_RL .* (Bx_RL .* kappa_x_RL - atan(Bx_RL .* kappa_x_RL)))) + S_Vx_RL; % will later be used in combined slip equations
    Fx0_RR = Dx_RR .* sin(Cx .* atan(Bx_RR .* kappa_x_RR - Ex_RR .* (Bx_RR .* kappa_x_RR - atan(Bx_RR .* kappa_x_RR)))) + S_Vx_RR; % will later be used in combined slip equations

    %% lateral (pure slip)
    % equations from Delft MF-Tyre User Manual Version 5.2
    % page 24 - 26
    Cy = p_Cy1;

    mu_y_FL = (p_Dy1 + p_Dy2 .* dfz_FL) .* (1-p_Dy3 .* gamma_FL.^2);
    mu_y_FR = (p_Dy1 + p_Dy2 .* dfz_FR) .* (1-p_Dy3 .* gamma_FR.^2);
    mu_y_RL = (p_Dy1 + p_Dy2 .* dfz_RL) .* (1-p_Dy3 .* gamma_RL.^2);
    mu_y_RR = (p_Dy1 + p_Dy2 .* dfz_RR) .* (1-p_Dy3 .* gamma_RR.^2);

    Dy_FL = mu_y_FL .* Fz_FL;
    Dy_FR = mu_y_FR .* Fz_FR;
    Dy_RL = mu_y_RL .* Fz_RL;
    Dy_RR = mu_y_RR .* Fz_RR;
    
    S_Hy_FL = p_Hy1 + p_Hy2 .* dfz_FL + p_Hy3 .* gamma_FL;
    S_Hy_FR = p_Hy1 + p_Hy2 .* dfz_FR + p_Hy3 .* gamma_FR;
    S_Hy_RL = p_Hy1 + p_Hy2 .* dfz_RL + p_Hy3 .* gamma_RL;
    S_Hy_RR = p_Hy1 + p_Hy2 .* dfz_RR + p_Hy3 .* gamma_RR;

    S_Vy_FL = Fz_FL .* (p_Vy1 + p_Vy2 .* dfz_FL + (p_Vy3 + p_Vy4 .* dfz_FL) .* gamma_FL);
    S_Vy_FR = Fz_FR .* (p_Vy1 + p_Vy2 .* dfz_FR + (p_Vy3 + p_Vy4 .* dfz_FR) .* gamma_FR);
    S_Vy_RL = Fz_RL .* (p_Vy1 + p_Vy2 .* dfz_RL + (p_Vy3 + p_Vy4 .* dfz_RL) .* gamma_RL);
    S_Vy_RR = Fz_RR .* (p_Vy1 + p_Vy2 .* dfz_RR + (p_Vy3 + p_Vy4 .* dfz_RR) .* gamma_RR);
    
    alpha_y_FL = slip_ang_FL + S_Hy_FL;
    alpha_y_FR = slip_ang_FR + S_Hy_FR;
    alpha_y_RL = slip_ang_RL + S_Hy_RL;
    alpha_y_RR = slip_ang_RR + S_Hy_RR;
    
    Ey_FL = (p_Ey1 + p_Ey2 .* dfz_FL) .* (1 - (p_Ey3 + p_Ey4 .* gamma_FL) .* sign(alpha_y_FL));
    Ey_FR = (p_Ey1 + p_Ey2 .* dfz_FR) .* (1 - (p_Ey3 + p_Ey4 .* gamma_FR) .* sign(alpha_y_FR));
    Ey_RL = (p_Ey1 + p_Ey2 .* dfz_RL) .* (1 - (p_Ey3 + p_Ey4 .* gamma_RL) .* sign(alpha_y_RL));
    Ey_RR = (p_Ey1 + p_Ey2 .* dfz_RR) .* (1 - (p_Ey3 + p_Ey4 .* gamma_RR) .* sign(alpha_y_RR));

    Ky_FL = p_Ky1 .* F_z0 .* sin(2 .* atan(Fz_FL ./ (p_Ky2 .* F_z0))) .* (1 - p_Ky3 .* abs(gamma_FL));
    Ky_FR = p_Ky1 .* F_z0 .* sin(2 .* atan(Fz_FR ./ (p_Ky2 .* F_z0))) .* (1 - p_Ky3 .* abs(gamma_FR));
    Ky_RL = p_Ky1 .* F_z0 .* sin(2 .* atan(Fz_RL ./ (p_Ky2 .* F_z0))) .* (1 - p_Ky3 .* abs(gamma_RL));
    Ky_RR = p_Ky1 .* F_z0 .* sin(2 .* atan(Fz_RR ./ (p_Ky2 .* F_z0))) .* (1 - p_Ky3 .* abs(gamma_RR));

    By_FL = Ky_FL / (Cy .* Dy_FL);
    By_FR = Ky_FR / (Cy .* Dy_FR);
    By_RL = Ky_RL / (Cy .* Dy_RL);
    By_RR = Ky_RR / (Cy .* Dy_RR);
    
    Fy0_FL = Dy_FL .* sin(Cy .* atan(By_FL .* alpha_y_FL - Ey_FL .* (By_FL .* alpha_y_FL - atan(By_FL .* alpha_y_FL)))) + S_Vy_FL; % will later be used in combined slip equations 
    Fy0_FR = Dy_FR .* sin(Cy .* atan(By_FR .* alpha_y_FR - Ey_FR .* (By_FR .* alpha_y_FR - atan(By_FR .* alpha_y_FR)))) + S_Vy_FR; % will later be used in combined slip equations 
    Fy0_RL = Dy_RL .* sin(Cy .* atan(By_RL .* alpha_y_RL - Ey_RL .* (By_RL .* alpha_y_RL - atan(By_RL .* alpha_y_RL)))) + S_Vy_RL; % will later be used in combined slip equations 
    Fy0_RR = Dy_RR .* sin(Cy .* atan(By_RR .* alpha_y_RR - Ey_RR .* (By_RR .* alpha_y_RR - atan(By_RR .* alpha_y_RR)))) + S_Vy_RR; % will later be used in combined slip equations 

    %% longitudinal (combined slip)
    % equations from Delft MF-Tyre User Manual Version 5.2
    % page 30 - 31
    S_Hxa = r_Hx1;

    alpha_s_FL = slip_ang_FL + S_Hxa;
    alpha_s_FR = slip_ang_FR + S_Hxa;
    alpha_s_RL = slip_ang_RL + S_Hxa;
    alpha_s_RR = slip_ang_RR + S_Hxa;
    
    Bxa_FL = r_Bx1 .* cos(atan(r_Bx2 .* long_slip_FL));
    Bxa_FR = r_Bx1 .* cos(atan(r_Bx2 .* long_slip_FR));
    Bxa_RL = r_Bx1 .* cos(atan(r_Bx2 .* long_slip_RL));
    Bxa_RR = r_Bx1 .* cos(atan(r_Bx2 .* long_slip_RR));

    Cxa = r_Cx1;

    Exa_FL = r_Ex1 + r_Ex2 .* dfz_FL;
    Exa_FR = r_Ex1 + r_Ex2 .* dfz_FR;
    Exa_RL = r_Ex1 + r_Ex2 .* dfz_RL;
    Exa_RR = r_Ex1 + r_Ex2 .* dfz_RR;
    
    Gxa_FL = (cos(Cxa .* atan(Bxa_FL .* alpha_s_FL - Exa_FL .* (Bxa_FL .* alpha_s_FL - atan(Bxa_FL .* alpha_s_FL))))) ./ ...
        (cos(Cxa .* atan(Bxa_FL .* S_Hxa - Exa_FL .* (Bxa_FL .* S_Hxa - atan(Bxa_FL .* S_Hxa)))));

    Gxa_FR = (cos(Cxa .* atan(Bxa_FR .* alpha_s_FR - Exa_FR .* (Bxa_FR .* alpha_s_FR - atan(Bxa_FR .* alpha_s_FR))))) ./ ...
        (cos(Cxa .* atan(Bxa_FR .* S_Hxa - Exa_FR .* (Bxa_FR .* S_Hxa - atan(Bxa_FR .* S_Hxa)))));
    
    Gxa_RL = (cos(Cxa .* atan(Bxa_RL .* alpha_s_RL - Exa_RL .* (Bxa_RL .* alpha_s_RL - atan(Bxa_RL .* alpha_s_RL))))) ./ ...
        (cos(Cxa .* atan(Bxa_RL .* S_Hxa - Exa_RL .* (Bxa_RL .* S_Hxa - atan(Bxa_RL .* S_Hxa)))));

    Gxa_RR = (cos(Cxa .* atan(Bxa_RR .* alpha_s_RR - Exa_RR .* (Bxa_RR .* alpha_s_RR - atan(Bxa_RR .* alpha_s_RR))))) ./ ...
        (cos(Cxa .* atan(Bxa_RR .* S_Hxa - Exa_RR .* (Bxa_RR .* S_Hxa - atan(Bxa_RR .* S_Hxa)))));
    
    Fx_FL = Fx0_FL .* Gxa_FL;
    Fx_FR = Fx0_FR .* Gxa_FR;
    Fx_RL = Fx0_RL .* Gxa_RL;
    Fx_RR = Fx0_RR .* Gxa_RR;

    %% lateral (combined slip)
    % equations from Delft MF-Tyre User Manual Version 5.2
    % page 32 - 33
    S_Hyk_FL = r_Hy1 + r_Hy2 .* dfz_FL;
    S_Hyk_FR = r_Hy1 + r_Hy2 .* dfz_FR;
    S_Hyk_RL = r_Hy1 + r_Hy2 .* dfz_RL;
    S_Hyk_RR = r_Hy1 + r_Hy2 .* dfz_RR;

    kappa_s_FL = long_slip_FL + S_Hyk_FL;
    kappa_s_FR = long_slip_FR + S_Hyk_FR;
    kappa_s_RL = long_slip_RL + S_Hyk_RL;
    kappa_s_RR = long_slip_RR + S_Hyk_RR;
    
    Byk_FL = r_By1 .* cos(atan(r_By2 .* (slip_ang_FL - r_By3)));
    Byk_FR = r_By1 .* cos(atan(r_By2 .* (slip_ang_FR - r_By3)));
    Byk_RL = r_By1 .* cos(atan(r_By2 .* (slip_ang_RL - r_By3)));
    Byk_RR = r_By1 .* cos(atan(r_By2 .* (slip_ang_RR - r_By3)));

    Cyk = r_Cy1;

    Eyk_FL = r_Ey1 + r_Ey2 .* dfz_FL;
    Eyk_FR = r_Ey1 + r_Ey2 .* dfz_FR;
    Eyk_RL = r_Ey1 + r_Ey2 .* dfz_RL;
    Eyk_RR = r_Ey1 + r_Ey2 .* dfz_RR;
    
    D_Vyk_FL = mu_y_FL .* Fz_FL .* (r_Vy1 + r_Vy2 .* dfz_FL + r_Vy3 .* gamma_FL) .* cos(atan(r_Vy4 .* slip_ang_FL));
    D_Vyk_FR = mu_y_FR .* Fz_FR .* (r_Vy1 + r_Vy2 .* dfz_FR + r_Vy3 .* gamma_FR) .* cos(atan(r_Vy4 .* slip_ang_FR));
    D_Vyk_RL = mu_y_RL .* Fz_RL .* (r_Vy1 + r_Vy2 .* dfz_RL + r_Vy3 .* gamma_RL) .* cos(atan(r_Vy4 .* slip_ang_RL));
    D_Vyk_RR = mu_y_RR .* Fz_RR .* (r_Vy1 + r_Vy2 .* dfz_RR + r_Vy3 .* gamma_RR) .* cos(atan(r_Vy4 .* slip_ang_RR));

    S_Vyk_FL = D_Vyk_FL .* sin(r_Vy5 .* atan(r_Vy6 .* long_slip_FL));
    S_Vyk_FR = D_Vyk_FR .* sin(r_Vy5 .* atan(r_Vy6 .* long_slip_FR));
    S_Vyk_RL = D_Vyk_RL .* sin(r_Vy5 .* atan(r_Vy6 .* long_slip_RL));
    S_Vyk_RR = D_Vyk_RR .* sin(r_Vy5 .* atan(r_Vy6 .* long_slip_RR));
    
    Gyk_FL = (cos(Cyk .* atan(Byk_FL .* kappa_s_FL - Eyk_FL .* (Byk_FL .* kappa_s_FL - atan(Byk_FL .* kappa_s_FL))))) ./ ...
        (cos(Cyk .* atan(Byk_FL .* S_Hyk_FL - Eyk_FL .* (Byk_FL .* S_Hyk_FL - atan(Byk_FL .* S_Hyk_FL)))));

    Gyk_FR = (cos(Cyk .* atan(Byk_FR .* kappa_s_FR - Eyk_FR .* (Byk_FR .* kappa_s_FR - atan(Byk_FR .* kappa_s_FR))))) ./ ...
        (cos(Cyk .* atan(Byk_FR .* S_Hyk_FR - Eyk_FR .* (Byk_FR .* S_Hyk_FR - atan(Byk_FR .* S_Hyk_FR)))));
    
    Gyk_RL = (cos(Cyk .* atan(Byk_RL .* kappa_s_RL - Eyk_RL .* (Byk_RL .* kappa_s_RL - atan(Byk_RL .* kappa_s_RL))))) ./ ...
        (cos(Cyk .* atan(Byk_RL .* S_Hyk_RL - Eyk_RL .* (Byk_RL .* S_Hyk_RL - atan(Byk_RL .* S_Hyk_RL)))));
    
    Gyk_RR = (cos(Cyk .* atan(Byk_RR .* kappa_s_RR - Eyk_RR .* (Byk_RR .* kappa_s_RR - atan(Byk_RR .* kappa_s_RR))))) ./ ...
        (cos(Cyk .* atan(Byk_RR .* S_Hyk_RR - Eyk_RR .* (Byk_RR .* S_Hyk_RR - atan(Byk_RR .* S_Hyk_RR)))));
    
    Fy_FL = Fy0_FL .* Gyk_FL + S_Vyk_FL; Fy_FL(isnan(Fy_FL)) = 0;
    Fy_FR = Fy0_FR .* Gyk_FR + S_Vyk_FR; Fy_FR(isnan(Fy_FR)) = 0;
    Fy_RL = Fy0_RL .* Gyk_RL + S_Vyk_RL; Fy_RL(isnan(Fy_RL)) = 0;
    Fy_RR = Fy0_RR .* Gyk_RR + S_Vyk_RR; Fy_RR(isnan(Fy_RR)) = 0;

    %% outputs
    Fx = [Fx_FL, Fx_FR, Fx_RL, Fx_RR];
    Fy = [Fy_FL, Fy_FR, Fy_RL, Fy_RR];

== matlab function tyre/slip_calculation/slip_states_mf52 ==
  data: v input; kappa output size=[1 4]; psi_p input; beta input; delta input; omega input; gamma input size=[1 4]; Fz input size=[1 4]; u input; w input; is_transient input; alpha output size=[1 4]; tire parameter; u_p output size=[1 4]; w_p output size=[1 4]; lF parameter; lR parameter; trackwidth_R parameter; trackwidth_F parameter
function [kappa, alpha, u_p, w_p]= fcn(v, psi_p, beta, delta, omega, gamma, Fz, u, w, is_transient, tire, lF, lR, trackwidth_R, trackwidth_F)
    %% parameters
    % vertical
    F_z0 = tire.Vertical.FNOMIN;
    c_z = tire.Vertical.VERTICAL_STIFFNESS;
    
    b_reff = tire.Vertical.BREFF;
    d_reff = tire.Vertical.DREFF;
    f_reff = tire.Vertical.FREFF;
    
    % dimension
    r_0 = tire.Dim.UNLOADED_RADIUS;

    % longitudinal (transient)
    p_Tx1 = tire.Long.PTX1;
    p_Tx2 = tire.Long.PTX2;
    p_Tx3 = tire.Long.PTX3;

    % lateral (transient)
    p_Ty1 = tire.Lat.PTY1;
    p_Ty2 = tire.Lat.PTY2;

    % lateral (pure slip)
    p_Ky3 = tire.Lat.PKY3;

    %% wheel steering angle mapping
    delta_FL = delta(1);
    delta_FR = delta(2);
    delta_RL = delta(3);
    delta_RR = delta(4);

    %% wheel rotational velocity mapping
    omega_FL = omega(1);
    omega_FR = omega(2);
    omega_RL = omega(3);
    omega_RR = omega(4);

    %% current camber mapping
    gamma_FL = gamma(1);
    gamma_FR = gamma(2);
    gamma_RL = gamma(3);
    gamma_RR = gamma(4);

    %% vertical load mapping
    Fz_FL = Fz(1);
    Fz_FR = Fz(2);
    Fz_RL = Fz(3);
    Fz_RR = Fz(4);

    %% longitudinal tyre deflection mapping
    u_FL = min(max(u(1), -0.01), 0.01);
    u_FR = min(max(u(2), -0.01), 0.01);
    u_RL = u(3);
    u_RR = u(4);

    %% lateral tyre deflection mapping
    w_FL = w(1);
    w_FR = w(2);
    w_RL = w(3);
    w_RR = w(4);

    %% effective rolling radius r_e
    % equations from Delft MF-Tyre User Manual Version 5.2
    % page 9 - 11
    p_FL = Fz_FL ./ c_z;
    p_FR = Fz_FR ./ c_z;
    p_RL = Fz_RL ./ c_z;
    p_RR = Fz_RR ./ c_z;
    
    p_Fz0 = F_z0 ./ c_z;
    
    p_d_FL = p_FL ./ p_Fz0;
    p_d_FR = p_FR ./ p_Fz0;
    p_d_RL = p_RL ./ p_Fz0;
    p_d_RR = p_RR ./ p_Fz0;
    
    r_e_FL = r_0 - (p_Fz0 .* (f_reff .* p_d_FL + d_reff .* atan(b_reff .* p_d_FL)));
    r_e_FR = r_0 - (p_Fz0 .* (f_reff .* p_d_FR + d_reff .* atan(b_reff .* p_d_FR)));
    r_e_RL = r_0 - (p_Fz0 .* (f_reff .* p_d_RL + d_reff .* atan(b_reff .* p_d_RL)));
    r_e_RR = r_0 - (p_Fz0 .* (f_reff .* p_d_RR + d_reff .* atan(b_reff .* p_d_RR)));
    
    %% velocity states
    % equation herritage not clear
    v_xFL = v .* cos(beta) - psi_p .* (trackwidth_F ./ 2);
    v_xFR = v .* cos(beta) + psi_p .* (trackwidth_F ./ 2);
    v_xRL = v .* cos(beta) - psi_p .* (trackwidth_R ./ 2);
    v_xRR = v .* cos(beta) + psi_p .* (trackwidth_F ./ 2);
    
    v_yFL = v .* sin(beta) + psi_p .* lF;
    v_yFR = v .* sin(beta) + psi_p .* lF;
    v_yRL = v .* sin(beta) - psi_p .* lR;
    v_yRR = v .* sin(beta) - psi_p .* lR;
    
    % vx in tire coordinate system 
    v_lon_FL = v_xFL .* cos(delta_FL) + v_yFL .* sin(delta_FL);
    v_lon_FR = v_xFR .* cos(delta_FR) + v_yFR .* sin(delta_FR);
    v_lon_RL = v_xRL .* cos(delta_RL) + v_yRL .* sin(delta_RL);
    v_lon_RR = v_xRR .* cos(delta_RR) + v_yRR .* sin(delta_RR);
    
    v_lat_FL = v_xFL .* sin(delta_FL) - v_yFL .* cos(delta_FL);
    v_lat_FR = v_xFR .* sin(delta_FR) - v_yFR .* cos(delta_FR);
    v_lat_RL = v_xRL .* sin(delta_RL) - v_yRL .* cos(delta_RL);
    v_lat_RR = v_xRR .* sin(delta_RR) - v_yRR .* cos(delta_RR);
    
    %% normalized vertical load
    % equations from Delft MF-Tyre User Manual Version 5.2
    % page 17
    dfz_FL = (Fz_FL - F_z0) ./ F_z0;
    dfz_FR = (Fz_FR - F_z0) ./ F_z0; 
    dfz_RL = (Fz_RL - F_z0) ./ F_z0; 
    dfz_RR = (Fz_RR - F_z0) ./ F_z0;
    
    %% longitudinal slip - kappa
    % equations from Delft MF-Tyre User Manual Version 5.2
    % page 12
    v_sx_FL = v_lon_FL - omega_FL .* r_e_FL;
    v_sx_FR = v_lon_FR - omega_FR .* r_e_FR;
    v_sx_RL = v_lon_RL - omega_RL .* r_e_RL;
    v_sx_RR = v_lon_RR - omega_RR .* r_e_RR;

    if is_transient
        % relaxation length
        sigma_k_FL = Fz_FL .* (p_Tx1 + p_Tx2 .* dfz_FL) .* exp(-p_Tx3 .* dfz_FL) .* (r_0 ./ F_z0);
        sigma_k_FR = Fz_FR .* (p_Tx1 + p_Tx2 .* dfz_FR) .* exp(-p_Tx3 .* dfz_FR) .* (r_0 ./ F_z0);
        sigma_k_RL = Fz_RL .* (p_Tx1 + p_Tx2 .* dfz_RL) .* exp(-p_Tx3 .* dfz_RL) .* (r_0 ./ F_z0);
        sigma_k_RR = Fz_RR .* (p_Tx1 + p_Tx2 .* dfz_RR) .* exp(-p_Tx3 .* dfz_RR) .* (r_0 ./ F_z0);

        u_p_FL = -v_sx_FL - (abs(v_lon_FL) ./ sigma_k_FL) .* u_FL;
        u_p_FR = -v_sx_FR - (abs(v_lon_FR) ./ sigma_k_FR) .* u_FR;
        u_p_RL = -v_sx_RL - (abs(v_lon_RL) ./ sigma_k_RL) .* u_RL;
        u_p_RR = -v_sx_RR - (abs(v_lon_RR) ./ sigma_k_RR) .* u_RR;

        long_slip_FL = (u_FL ./ sigma_k_FL) .* sign(v_lon_FL); if isnan(long_slip_FL); long_slip_FL = - v_sx_FL ./ v_lon_FL; end % switch to non transient if Fz not defined
        long_slip_FR = (u_FR ./ sigma_k_FR) .* sign(v_lon_FR); if isnan(long_slip_FR); long_slip_FR = - v_sx_FR ./ v_lon_FR; end % switch to non transient if Fz not defined
        long_slip_RL = (u_RL ./ sigma_k_RL) .* sign(v_lon_RL); if isnan(long_slip_RL); long_slip_RL = - v_sx_RL ./ v_lon_RL; end % switch to non transient if Fz not defined
        long_slip_RR = (u_RR ./ sigma_k_RR) .* sign(v_lon_RR); if isnan(long_slip_RR); long_slip_RR = - v_sx_RR ./ v_lon_RR; end % switch to non transient if Fz not defined
    else
        long_slip_FL = - v_sx_FL ./ v_lon_FL;
        long_slip_FR = - v_sx_FR ./ v_lon_FR;
        long_slip_RL = - v_sx_RL ./ v_lon_RL;
        long_slip_RR = - v_sx_RR ./ v_lon_RR;

        u_p_FL = 0;
        u_p_FR = 0;
        u_p_RL = 0;
        u_p_RR = 0;
    end

    %% slip angle - alpha
    % effektiver Lenkwinkel
    delta_eff_FL = atan(v_yFL ./ v_xFL);
    delta_eff_FR = atan(v_yFR ./ v_xFR);
    delta_eff_RL = atan(v_yRL ./ v_xRL);
    delta_eff_RR = atan(v_yRR ./ v_xRR);
    
    if is_transient
        sigma_a_FL = p_Ty1 .* sin(2.*atan(Fz_FL ./ (p_Ty2 .* F_z0))) .* (1 - p_Ky3 .* abs(gamma_FL)) .* r_0;
        sigma_a_FR = p_Ty1 .* sin(2.*atan(Fz_FR ./ (p_Ty2 .* F_z0))) .* (1 - p_Ky3 .* abs(gamma_FR)) .* r_0;
        sigma_a_RL = p_Ty1 .* sin(2.*atan(Fz_RL ./ (p_Ty2 .* F_z0))) .* (1 - p_Ky3 .* abs(gamma_RL)) .* r_0;
        sigma_a_RR = p_Ty1 .* sin(2.*atan(Fz_RR ./ (p_Ty2 .* F_z0))) .* (1 - p_Ky3 .* abs(gamma_RR)) .* r_0;

        w_p_FL = v_lat_FL - (abs(v_lon_FL) ./ sigma_a_FL) .* w_FL;
        w_p_FR = v_lat_FR - (abs(v_lon_FR) ./ sigma_a_FR) .* w_FR;
        w_p_RL = v_lat_RL - (abs(v_lon_RL) ./ sigma_a_RL) .* w_RL;
        w_p_RR = v_lat_RR - (abs(v_lon_RR) ./ sigma_a_RR) .* w_RR;

        slip_ang_FL = -atan(w_FL ./ sigma_a_FL); if isnan(slip_ang_FL); slip_ang_FL = 0; end % switch to non transient if Fz not defined
        slip_ang_FR = -atan(w_FR ./ sigma_a_FR); if isnan(slip_ang_FR); slip_ang_FR = 0; end % switch to non transient if Fz not defined
        slip_ang_RL = -atan(w_RL ./ sigma_a_RL); if isnan(slip_ang_RL); slip_ang_RL = 0; end % switch to non transient if Fz not defined
        slip_ang_RR = -atan(w_RR ./ sigma_a_RR); if isnan(slip_ang_RR); slip_ang_RR = 0; end % switch to non transient if Fz not defined

    else
        slip_ang_FL = -(delta_FL - delta_eff_FL);
        slip_ang_FR = -(delta_FR - delta_eff_FR);
        slip_ang_RL = -(delta_RL - delta_eff_RL);
        slip_ang_RR = -(delta_RR - delta_eff_RR);

        w_p_FL = 0;
        w_p_FR = 0;
        w_p_RL = 0;
        w_p_RR = 0;
    end

    %% outputs
    kappa = [long_slip_FL, long_slip_FR, long_slip_RL, long_slip_RR];
    alpha = [slip_ang_FL, slip_ang_FR, slip_ang_RL, slip_ang_RR];
    
    u_p   = [u_p_FL, u_p_FR, u_p_RL, u_p_RR];
    w_p   = [w_p_FL, w_p_FR, w_p_RL, w_p_RR];
